simulink model "test_fmu_v2"  (R2022a)
settings: Solver=FixedStepAuto  StartTime=0.0  StopTime=10.0  RelTol=1e-3
settings Model: Creator=lordx  LastModifiedBy=lordx
settings RTWCC: Description=FMU based on GRT (Functional Mock-up Unit)  SystemTargetFile=grtfmi.tlc  GenerateMakefile=off  TemplateMakefile=none  GenerateReport=on  RetainRTWFile=on
settings CodeAppCC: ForceParamTrailComments=on  StateflowObjectComments=on  MATLABSourceComments=on
settings STFCustomTargetCC: TargetLangStandard=C99 (ISO)  CombineOutputUpdateFcns=on  GRTInterface=off  OptimizeReductions=on  SystemTargetFile=grtfmi.tlc
settings GRTTargetCC: ParMdlRefBuildCompliant=off  CompOptLevelCompliant=off  ConcurrentExecutionCompliant=off  MatFileLogging=off  CPPClassGenCompliant=off  UseToolchainInfoCompliant=off  OptimizeReductions=on  RTWCAPISignals=on  RTWCAPIParams=on  RTWCAPIStates=on  RTWCAPIRootIO=on

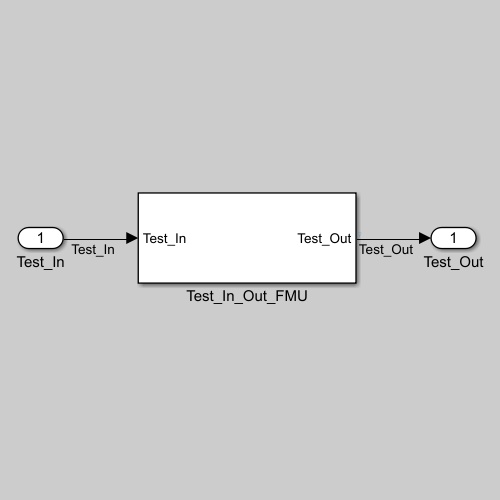
[thumbnail: Simulink's stored preview of the top-level diagram]
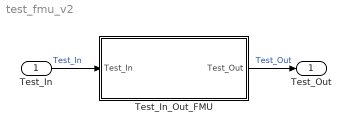
== system test_fmu_v2 ==
  Test_In : Inport
  Test_In_Out_FMU : Subsystem
  Test_Out : Outport
  wires:
  Test_In/1 -> Test_In_Out_FMU/1(Test_In)  "Test_In"
  Test_In_Out_FMU/1(Test_Out) -> Test_Out/1  "Test_Out"

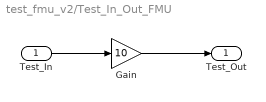
== system test_fmu_v2/Test_In_Out_FMU ==
  Test_In : Inport
  Gain : Gain  Gain=10
  Test_Out : Outport
  wires:
  Test_In/1 -> Gain/1
  Gain/1 -> Test_Out/1
